simulink library "INT_Conv_LdCalc"  (R2016b)
settings: Solver=VariableStepAuto  StartTime=0.0  StopTime=10.0  RelTol=1e-3
settings Model: Creator=Administrator  LastModifiedBy=Administrator

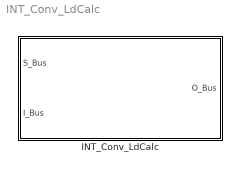
== system INT_Conv_LdCalc ==
  INT_Conv_LdCalc : Subsystem

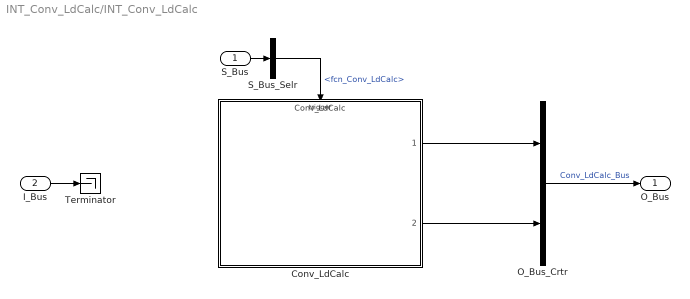
== system INT_Conv_LdCalc/INT_Conv_LdCalc ==
  S_Bus : Inport
  I_Bus : Inport  Port=2
  Conv_LdCalc : ModelReference  ModelNameDialog=Conv_LdCalc  SimulationMode=Normal  ModelReferenceVersion=1.2  TriggerPortName=function  TriggerPortTriggerType=function-call  TriggerPortStatesWhenEnabling=held
  O_Bus_Crtr : BusCreator  Inputs=2
  S_Bus_Selr : BusSelector  OutputSignals=fcn_Conv_LdCalc
  Terminator : Terminator
  O_Bus : Outport
  wires:
  S_Bus_Selr/1 -> Conv_LdCalc/Trigger  "<fcn_Conv_LdCalc>"
  S_Bus/1 -> S_Bus_Selr/1
  I_Bus/1 -> Terminator/1
  O_Bus_Crtr/1 -> O_Bus/1  "Conv_LdCalc_Bus"
  Conv_LdCalc/1 -> O_Bus_Crtr/1
  Conv_LdCalc/2 -> O_Bus_Crtr/2
